simulink model "diferencia"  (R2022a)
settings: Solver=VariableStepAuto  StartTime=0.0  StopTime=inf  RelTol=1e-3
undefined symbols (not defined in the file): none, Rec, SDTV, videoinput
libraries: visionconversions x1, simulink x1, visiontextngfix x1, imaqlib x1
settings Model: Creator=misog  LastModifiedBy=misog

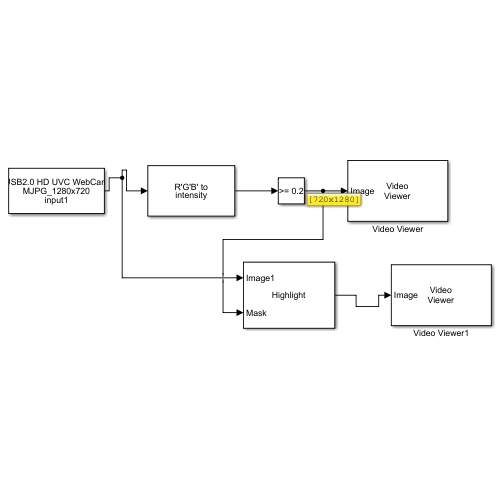
[thumbnail: Simulink's stored preview of the top-level diagram]
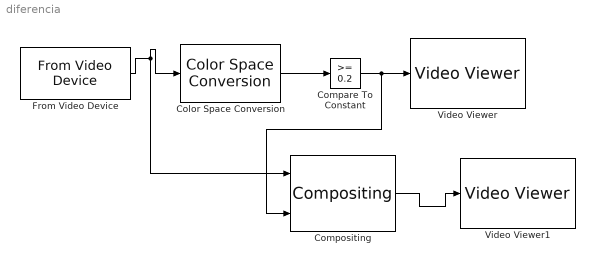
== system diferencia ==
  Color Space Conversion : visionconversions/Color Space  Conversion  conversion=Obsolete  conversionActive=R'G'B' to intensity  wp_str=D65  rec=Rec. 601 (SDTV)  sys=1125/60/2:1  imagePorts=One multidimensional signal
  Compare To Constant : simulink/Logic and Bit Operations/Compare To Constant  relop=>=  const=0.2  OutDataTypeStr=boolean  ZeroCross=off
  Compositing : visiontextngfix/Compositing  operation=Highlight selected pixels  bFacSrc=Specify via dialog  bFactor=0.05  mFacSrc=Specify via dialog  mFactor=1  source=Specify via dialog  coordinates=[1 1]  roundingMode=Floor  overflowMode=off  prodOutputMode=Binary point scaling  prodOutputWordLength=32  prodOutputFracLength=10
      settings: SourceProductBaseCode=VP
  From Video Device : imaqlib/From Video Device  DeviceMenu=winvideo 1 (USB2.0 HD UVC WebCam)  Device=winvideo 1 (USB2.0 HD UVC WebCam)  ObjConstructor=videoinput('winvideo', 1)  VideoFormatMenu=MJPG_1280x720  VideoFormat=MJPG_1280x720  VideoSource=input1  ROIPosition=[0 0 720 1280]  EnableHWTrigger=off  TriggerConfiguration=none/none  SampleTime=1/30  OutputPortsMode=One multidimensional signal  DataType=single  CanDoHWTrigger=no  ReturnedColorSpace=rgb  BlockHandle=4.0004  ROIWidth=1280  ROIHeight=720  ROIColumn=0  ROIRow=0  EngXMLPath=C:\Program Files\MATLAB\R2022a\toolbox\imaq\imaq\private  DevXMLPath=C:\ProgramData\MATLAB\SupportPackages\R2022a\toolbox\imaq\supportpackages\genericvideo\adaptor\win64  EngLibPath=C:\Program Files\MATLAB\R2022a\toolbox\imaq\imaqblks\imaqmex\win64  ColorSpace=rgb  BayerSensorAlignment=grbg  ImaqMode=off
  Video Viewer : VideoViewer  FigPos=[2 1077 958 969]
  Video Viewer1 : VideoViewer  FigPos=[962 1077 958 969]
  wires:
  From Video Device/1 -> Compositing/1, Color Space Conversion/1
  Color Space Conversion/1 -> Compare To Constant/1
  Compare To Constant/1 -> Compositing/2, Video Viewer/1
  Compositing/1 -> Video Viewer1/1
